simulink model "SystemLoopDiscreteBeuti"  (R2023a)
settings: Solver=VariableStepAuto  StartTime=0.0  StopTime=50  RelTol=1e-3
values from neighbouring files (symbols this model uses):
  L = 8.2*10^(-3)    (= 0.0082)    [phaseplane.m]
undefined symbols (not defined in the file or in its folder): Ad, Bd, Cd, Dd, DiscIntNeverNeededParam, ki, Kp, Ts
libraries: mbedblockslib x3, cstblocks x1, stm_qeplib x1
settings Model: Creator=Marco  LastModifiedBy=Marco

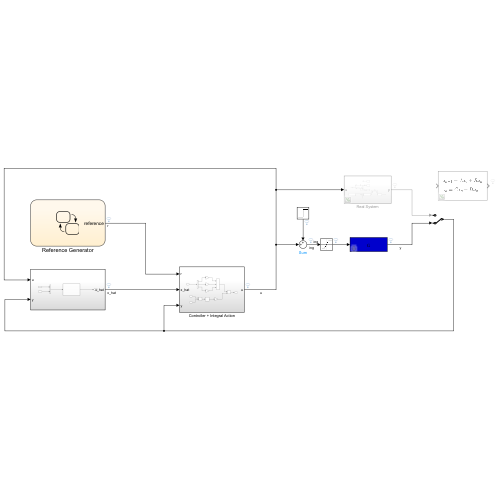
[thumbnail: Simulink's stored preview of the top-level diagram]
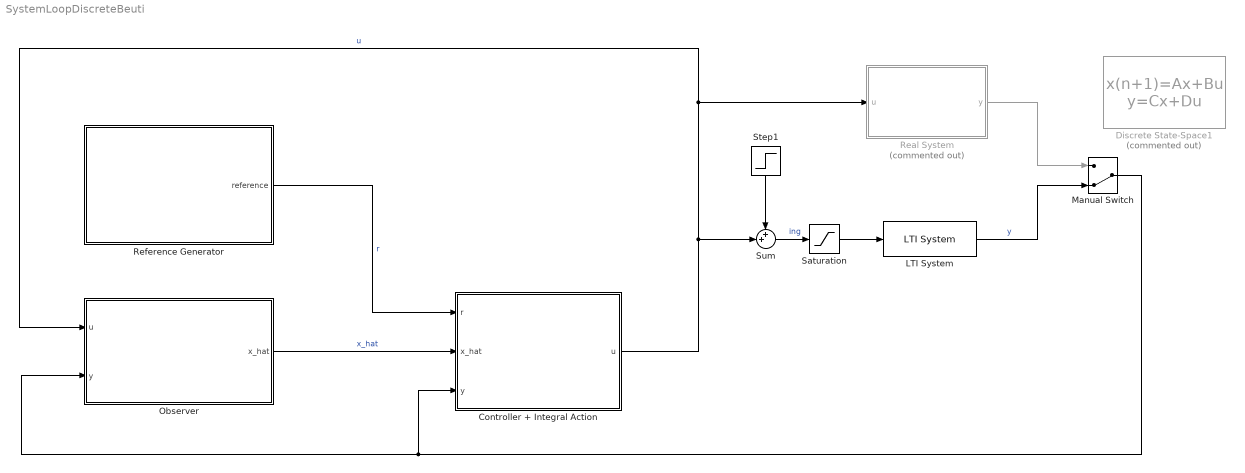
== system SystemLoopDiscreteBeuti ==
  Controller + Integral Action : Subsystem
  Discrete State-Space1 : DiscreteStateSpace  Commented=on  A=Ad  B=Bd  C=Cd  D=Dd  SampleTime=Ts
  LTI System : cstblocks/LTI System  sys=G  IC=[]
  Manual Switch : ManualSwitch  CurrentSetting=0
  Observer : Subsystem
  Real System : Subsystem  Commented=on
  Reference Generator : Stateflow chart  TreatAsAtomicUnit=on
  Saturation : Saturate  UpperLimit=12  LowerLimit=-12
  Step1 : Step  Time=3  After=1.2  SampleTime=Ts
  Sum : Sum  Inputs=++|
  wires:
  Reference Generator/1(reference) -> Controller + Integral Action/1(r)  "r"
  Controller + Integral Action/1(u) -> Sum/2, Real System/1(u), Observer/1(u)  "u"
  Real System/1(y) -> Manual Switch/1
  LTI System/1 -> Manual Switch/2  "y"
  Manual Switch/1 -> Controller + Integral Action/3(y), Observer/2(y)
  Observer/1(x_hat) -> Controller + Integral Action/2(x_hat)  "x_hat"
  Sum/1 -> Saturation/1  "ing"
  Step1/1 -> Sum/1
  Saturation/1 -> LTI System/1

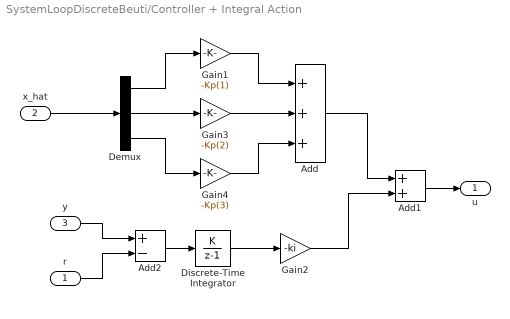
== system SystemLoopDiscreteBeuti/Controller + Integral Action ==
  r : Inport
  x_hat : Inport  Port=2
  y : Inport  Port=3
  Add : Sum  Inputs=+++
  Add1 : Sum
  Add2 : Sum  Inputs=+-
  Demux : Demux  Outputs=3
  Discrete-Time Integrator : DiscreteIntegrator  IntegratorMethod=Accumulation: Forward Euler  gainval=1  SampleTime=Ts  StateName='IntegralAction'  ICPrevOutput=DiscIntNeverNeededParam  ICPrevScaledInput=DiscIntNeverNeededParam
  Gain1 : Gain  Gain=-Kp(1)
  Gain2 : Gain  Gain=-ki
  Gain3 : Gain  Gain=-Kp(2)
  Gain4 : Gain  Gain=-Kp(3)
  u : Outport
  wires:
  r/1 -> Add2/2
  Add2/1 -> Discrete-Time Integrator/1
  y/1 -> Add2/1
  Discrete-Time Integrator/1 -> Gain2/1
  Demux/2 -> Gain3/1
  x_hat/1 -> Demux/1
  Demux/3 -> Gain4/1
  Demux/1 -> Gain1/1
  Gain1/1 -> Add/1
  Add/1 -> Add1/1
  Gain4/1 -> Add/3
  Gain3/1 -> Add/2
  Add1/1 -> u/1
  Gain2/1 -> Add1/2

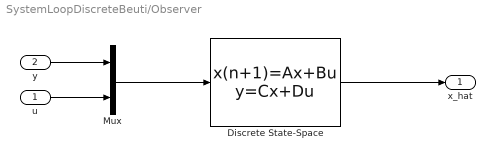
== system SystemLoopDiscreteBeuti/Observer ==
  u : Inport
  y : Inport  Port=2
  Discrete State-Space : DiscreteStateSpace  A=Ad-L*Cd  B=[Bd L]  C=eye(3)  D=[ 0 0; 0 0; 0 0]  SampleTime=Ts
  Mux : Mux  Inputs=2
  x_hat : Outport
  wires:
  Discrete State-Space/1 -> x_hat/1
  Mux/1 -> Discrete State-Space/1
  y/1 -> Mux/1
  u/1 -> Mux/2

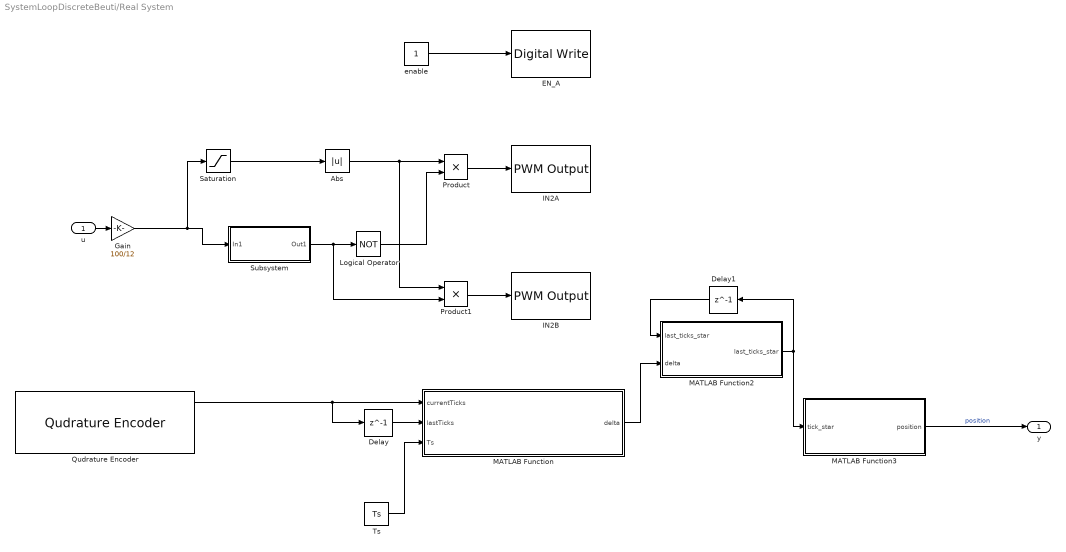
== system SystemLoopDiscreteBeuti/Real System ==
  u : Inport
  Abs : Abs  SaturateOnIntegerOverflow=off
  Delay : Delay  DelayLength=1  InitialCondition=0
  Delay1 : Delay  DelayLength=1  InitialCondition=0
  EN_A : mbedblockslib/Digital Write  Pin=2  Direction=output
      settings: LibrarySourceBlock=stmnucleorootlib/Common/Digital Write
  Gain : Gain  Gain=100/12
  IN2A : mbedblockslib/PWM Output  Pin=4  EnableInputFrequency=off  InitialFrequency=PWMFreq  InitialDutyCycle=50  NotificationType=None
      settings: LibrarySourceBlock=stmnucleorootlib/Common/PWM Output
  IN2B : mbedblockslib/PWM Output  Pin=5  EnableInputFrequency=off  InitialFrequency=PWMFreq  InitialDutyCycle=50  NotificationType=None
      settings: LibrarySourceBlock=stmnucleorootlib/Common/PWM Output
  Logical Operator : Logic  Operator=NOT  AllPortsSameDT=off  OutDataTypeStr=boolean
  MATLAB Function : MATLAB Function  TreatAsAtomicUnit=on
  MATLAB Function2 : MATLAB Function  TreatAsAtomicUnit=on
  MATLAB Function3 : MATLAB Function  TreatAsAtomicUnit=on
  Product : Product
  Product1 : Product
  Qudrature Encoder : stm_qeplib/Qudrature Encoder  SampleTime=Ts
  Saturation : Saturate  UpperLimit=100  LowerLimit=-100
  Subsystem : Subsystem
  Ts : Constant  Value=Ts
  enable : Constant
  y : Outport
  wires:
  enable/1 -> EN_A/1
  Subsystem/1(Out1) -> Product1/2, Logical Operator/1
  Saturation/1 -> Abs/1
  Product1/1 -> IN2B/1
  Product/1 -> IN2A/1
  Logical Operator/1 -> Product/2
  Abs/1 -> Product1/1, Product/1
  Gain/1 -> Saturation/1, Subsystem/1(In1)
  MATLAB Function2/1(last_ticks_star) -> MATLAB Function3/1(tick_star), Delay1/1
  Qudrature Encoder/1 -> Delay/1, MATLAB Function/1(currentTicks)
  MATLAB Function/1(delta) -> MATLAB Function2/2(delta)
  Delay1/1 -> MATLAB Function2/1("last_ticks_star ")
  Ts/1 -> MATLAB Function/3(Ts)
  Delay/1 -> MATLAB Function/2(lastTicks)
  u/1 -> Gain/1
  MATLAB Function3/1(position) -> y/1  "position"

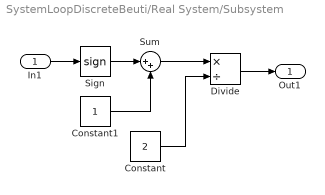
== system SystemLoopDiscreteBeuti/Real System/Subsystem ==
  In1 : Inport
  Constant : Constant  Value=2
  Constant1 : Constant
  Divide : Product  Inputs=*/
  Sign : Signum
  Sum : Sum  Inputs=|++
  Out1 : Outport
  wires:
  In1/1 -> Sign/1
  Sign/1 -> Sum/1
  Constant1/1 -> Sum/2
  Sum/1 -> Divide/1
  Constant/1 -> Divide/2
  Divide/1 -> Out1/1

== stateflow chart SystemLoopDiscreteBeuti/Reference Generator ==
  state Start
    reference = 0;
  state State1
    reference = deg2rad(180)
  state State4
    reference = deg2rad(-180)
  state State2
    reference = deg2rad(360)
  state State3
    reference = deg2rad(270)
  state State5
    reference = 0
  (default) -> Start
  Start -> State1 : [after(4,sec)]
  State1 -> State4 : [after(4,sec)]
  State4 -> State2 : [after(4,sec)]
  State3 -> Start : [after(4,sec)]
  State2 -> State5 : [after(4,sec)]
  State5 -> State3 : [after(4,sec)]
  data: reference output

== matlab function SystemLoopDiscreteBeuti/Real System/MATLAB Function ==
  data: currentTicks input; delta output; lastTicks input; Ts input
function delta = getTicksDelta(currentTicks, lastTicks, Ts)

currentTicks = double(currentTicks);
lastTicks = double(lastTicks);

if abs(currentTicks - lastTicks) <= ceil(8400*Ts)
    delta = currentTicks-lastTicks;
else
    if lastTicks > currentTicks
        delta = currentTicks + 2^16-1-lastTicks;
    else
        delta = currentTicks - 2^16+1-lastTicks;

end

end

== matlab function SystemLoopDiscreteBeuti/Real System/MATLAB Function2 ==
  data: last_ticks_star input; delta input; last_ticks_star output
function last_ticks_star = modCounter(last_ticks_star,delta)
     sum = last_ticks_star+delta;
	 last_ticks_star = sign(sum)*mod(abs(sum),89796);

end

== matlab function SystemLoopDiscreteBeuti/Real System/MATLAB Function3 ==
  data: tick_star input; position output
function position = getPosition(tick_star)

    ticks_star = double(tick_star);

    position = 2*pi*ticks_star/(3591.84);

end
